simulink model "controller"  (R2023b)
settings: Solver=VariableStepAuto  StartTime=0.0  StopTime=10.0  RelTol=1e-3
undefined symbols (not defined in the file): p
libraries: simulink x6
settings Model: Creator=kirill  LastModifiedBy=kirill

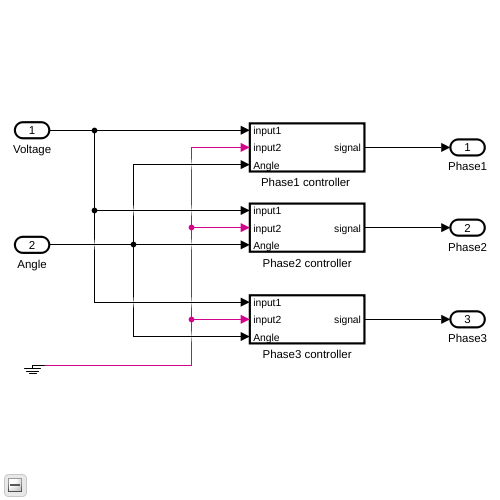
[thumbnail: Simulink's stored preview of the top-level diagram]
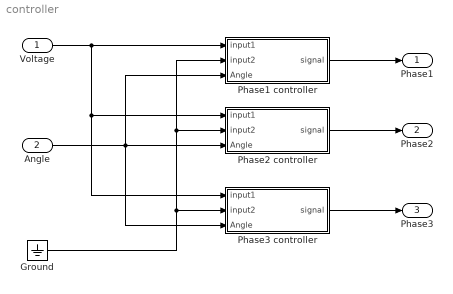
== system controller ==
  Voltage : Inport
  Angle : Inport  Port=2
  Ground : Ground
  "Phase1 controller " : Subsystem
  Phase2 controller : Subsystem
  Phase3 controller : Subsystem
  Phase1 : Outport
  Phase2 : Outport  Port=2
  Phase3 : Outport  Port=3
  wires:
  "Phase1 controller "/1(signal) -> Phase1/1
  Phase2 controller/1(signal) -> Phase2/1
  Phase3 controller/1(signal) -> Phase3/1
  Angle/1 -> Phase3 controller/3(Angle), Phase2 controller/3(Angle), "Phase1 controller "/3(Angle)
  Ground/1 -> Phase3 controller/2(input2), Phase2 controller/2(input2), "Phase1 controller "/2(input2)
  Voltage/1 -> "Phase1 controller "/1(input1), Phase3 controller/1(input1), Phase2 controller/1(input1)

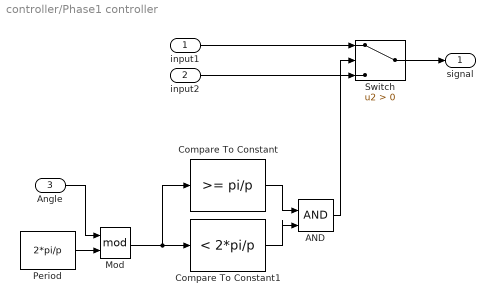
== system controller/Phase1 controller  ==
  input1 : Inport
  input2 : Inport  Port=2
  Angle : Inport  Port=3
  AND : Logic  IconShape=distinctive  AllPortsSameDT=off  OutDataTypeStr=boolean
  Compare To Constant : simulink/Logic and Bit Operations/Compare To Constant  relop=>=  const=pi/p  OutDataTypeStr=boolean
  Compare To Constant1 : simulink/Logic and Bit Operations/Compare To Constant  relop=<  const=2*pi/p  OutDataTypeStr=boolean
  Mod : Math  Operator=mod
  Period : Constant  Value=2*pi/p
  Switch : Switch  Criteria=u2 > Threshold  SaturateOnIntegerOverflow=off  InputSameDT=off
  signal : Outport
  wires:
  Angle/1 -> Mod/1
  Period/1 -> Mod/2
  Mod/1 -> Compare To Constant/1, Compare To Constant1/1
  Compare To Constant/1 -> AND/1
  Compare To Constant1/1 -> AND/2
  input1/1 -> Switch/1
  input2/1 -> Switch/3
  AND/1 -> Switch/2
  Switch/1 -> signal/1

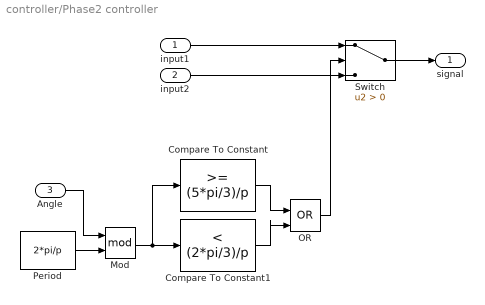
== system controller/Phase2 controller ==
  input1 : Inport
  input2 : Inport  Port=2
  Angle : Inport  Port=3
  Compare To Constant : simulink/Logic and Bit Operations/Compare To Constant  relop=>=  const=(5*pi/3)/p  OutDataTypeStr=boolean
  Compare To Constant1 : simulink/Logic and Bit Operations/Compare To Constant  relop=<  const=(2*pi/3)/p  OutDataTypeStr=boolean
  Mod : Math  Operator=mod
  OR : Logic  Operator=OR  IconShape=distinctive  AllPortsSameDT=off  OutDataTypeStr=boolean
  Period : Constant  Value=2*pi/p
  Switch : Switch  Criteria=u2 > Threshold  SaturateOnIntegerOverflow=off  InputSameDT=off
  signal : Outport
  wires:
  Switch/1 -> signal/1
  Compare To Constant/1 -> OR/1
  input1/1 -> Switch/1
  Period/1 -> Mod/2
  Mod/1 -> Compare To Constant/1, Compare To Constant1/1
  Compare To Constant1/1 -> OR/2
  input2/1 -> Switch/3
  OR/1 -> Switch/2
  Angle/1 -> Mod/1

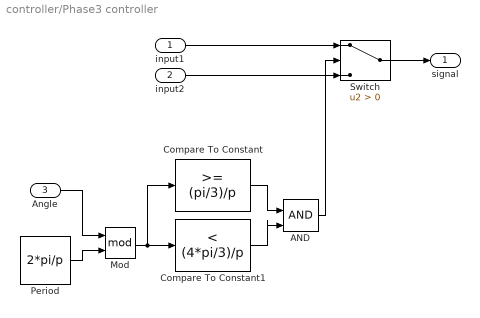
== system controller/Phase3 controller ==
  input1 : Inport
  input2 : Inport  Port=2
  Angle : Inport  Port=3
  AND : Logic  IconShape=distinctive  AllPortsSameDT=off  OutDataTypeStr=boolean
  Compare To Constant : simulink/Logic and Bit Operations/Compare To Constant  relop=>=  const=(pi/3)/p  OutDataTypeStr=boolean
  Compare To Constant1 : simulink/Logic and Bit Operations/Compare To Constant  relop=<  const=(4*pi/3)/p  OutDataTypeStr=boolean
  Mod : Math  Operator=mod
  Period : Constant  Value=2*pi/p
  Switch : Switch  Criteria=u2 > Threshold  SaturateOnIntegerOverflow=off  InputSameDT=off
  signal : Outport
  wires:
  Switch/1 -> signal/1
  Compare To Constant/1 -> AND/1
  input1/1 -> Switch/1
  Period/1 -> Mod/2
  Mod/1 -> Compare To Constant/1, Compare To Constant1/1
  Compare To Constant1/1 -> AND/2
  input2/1 -> Switch/3
  AND/1 -> Switch/2
  Angle/1 -> Mod/1
